simulink model "torqueBalancingSOT2017a"  (Simulink 8.9)
settings: Solver=FixedStepDiscrete  StartTime=0.0  StopTime=CONFIG.SIMULATION_TIME  FixedStep=CONFIG.Ts  RelTol=1e-3  EnableMultiTasking=on
InitFcn:
  | cd(fileparts(which(bdroot)));
  | initTorqueBalancingSOT;
undefined symbols (not defined in the file or in its folder): CONFIG, ConstraintsFeetMatrix, DiscIntNeverNeededParam, gain, reg, ROBOT_DOF, sat, sm, WBT_robotName
undefined symbols (not defined in the file): FRAMES
libraries: WBToolboxLibrary x76
(part 2 of 2)

== system torqueBalancingSOT2017a/Visualize and log/Visualize feet constraints ==
  wrench_leftFoot : Inport
  wrench_rightFoot : Inport  Port=2
  feetConstraints : Inport  Port=3
  state : Inport  Port=4
  Enable : EnablePort
  Feet Constraints : Scope  NumInputPorts=4
  wires:
  state/1 -> Feet Constraints/4  "state"
  feetConstraints/1 -> Feet Constraints/3  "feetConstraints"
  wrench_rightFoot/1 -> Feet Constraints/2  "wrench_rightFoot"
  wrench_leftFoot/1 -> Feet Constraints/1  "wrench_leftFoot"

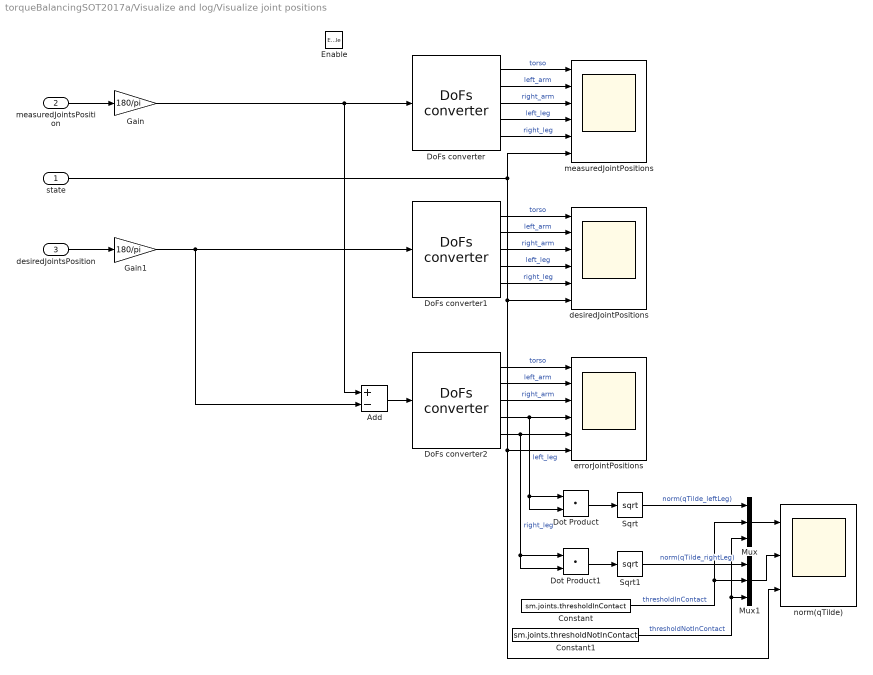
== system torqueBalancingSOT2017a/Visualize and log/Visualize joint positions ==
  state : Inport
  measuredJointsPosition : Inport  Port=2
  desiredJointsPosition : Inport  Port=3
  Enable : EnablePort
  Add : Sum  Inputs=+-
  Constant : Constant  Value=sm.joints.thresholdInContact
  Constant1 : Constant  Value=sm.joints.thresholdNotInContact
  DoFs converter : WBToolboxLibrary/Utilities/DoFs converter  yarp2WBIOption=From WBI to YARP  robotName=WBT_robotName  localName=WBT_modelName  wbiFile=WBT_wbiFilename  wbiList=WBT_wbiList
      settings: SourceProductName=Whole Body Toolbox
  DoFs converter1 : WBToolboxLibrary/Utilities/DoFs converter  yarp2WBIOption=From WBI to YARP  robotName=WBT_robotName  localName=WBT_modelName  wbiFile=WBT_wbiFilename  wbiList=WBT_wbiList
      settings: SourceProductName=Whole Body Toolbox
  DoFs converter2 : WBToolboxLibrary/Utilities/DoFs converter  yarp2WBIOption=From WBI to YARP  robotName=WBT_robotName  localName=WBT_modelName  wbiFile=WBT_wbiFilename  wbiList=WBT_wbiList
      settings: SourceProductName=Whole Body Toolbox
  Dot Product : DotProduct  InputSameDT=on  OutDataTypeStr=Inherit: Inherit via internal rule
  Dot Product1 : DotProduct  InputSameDT=on  OutDataTypeStr=Inherit: Inherit via internal rule
  Gain : Gain  Gain=180/pi
  Gain1 : Gain  Gain=180/pi
  Mux : Mux  Inputs=3
  Mux1 : Mux  Inputs=3
  Sqrt : Sqrt  SaturateOnIntegerOverflow=on
  Sqrt1 : Sqrt  SaturateOnIntegerOverflow=on
  desiredJointPositions : Scope  NumInputPorts=6
  errorJointPositions : Scope  NumInputPorts=6
  measuredJointPositions : Scope  NumInputPorts=6
  norm(qTilde) : Scope  NumInputPorts=3
  wires:
  DoFs converter/5 -> measuredJointPositions/5  "right_leg"
  DoFs converter/4 -> measuredJointPositions/4  "left_leg"
  DoFs converter/2 -> measuredJointPositions/2  "left_arm"
  DoFs converter/1 -> measuredJointPositions/1  "torso"
  DoFs converter2/2 -> errorJointPositions/2  "left_arm"
  DoFs converter2/1 -> errorJointPositions/1  "torso"
  desiredJointsPosition/1 -> Gain1/1
  measuredJointsPosition/1 -> Gain/1
  DoFs converter2/4 -> errorJointPositions/4, Dot Product/1, Dot Product/2  "left_leg"
  DoFs converter1/1 -> desiredJointPositions/1  "torso"
  DoFs converter1/3 -> desiredJointPositions/3  "right_arm"
  DoFs converter1/4 -> desiredJointPositions/4  "left_leg"
  Add/1 -> DoFs converter2/1
  Gain/1 -> Add/1, DoFs converter/1
  DoFs converter/3 -> measuredJointPositions/3  "right_arm"
  DoFs converter1/2 -> desiredJointPositions/2  "left_arm"
  DoFs converter2/3 -> errorJointPositions/3  "right_arm"
  DoFs converter2/5 -> errorJointPositions/5, Dot Product1/2, Dot Product1/1  "right_leg"
  DoFs converter1/5 -> desiredJointPositions/5  "right_leg"
  state/1 -> measuredJointPositions/6, norm(qTilde)/3, errorJointPositions/6, desiredJointPositions/6
  Dot Product/1 -> Sqrt/1
  Dot Product1/1 -> Sqrt1/1
  Sqrt/1 -> Mux/1  "norm(qTilde_leftLeg)"
  Sqrt1/1 -> Mux1/1  "norm(qTilde_rightLeg)"
  Constant/1 -> Mux/2, Mux1/2  "thresholdInContact"
  Constant1/1 -> Mux1/3, Mux/3  "thresholdNotInContact"
  Mux/1 -> norm(qTilde)/1
  Mux1/1 -> norm(qTilde)/2
  Gain1/1 -> Add/2, DoFs converter1/1

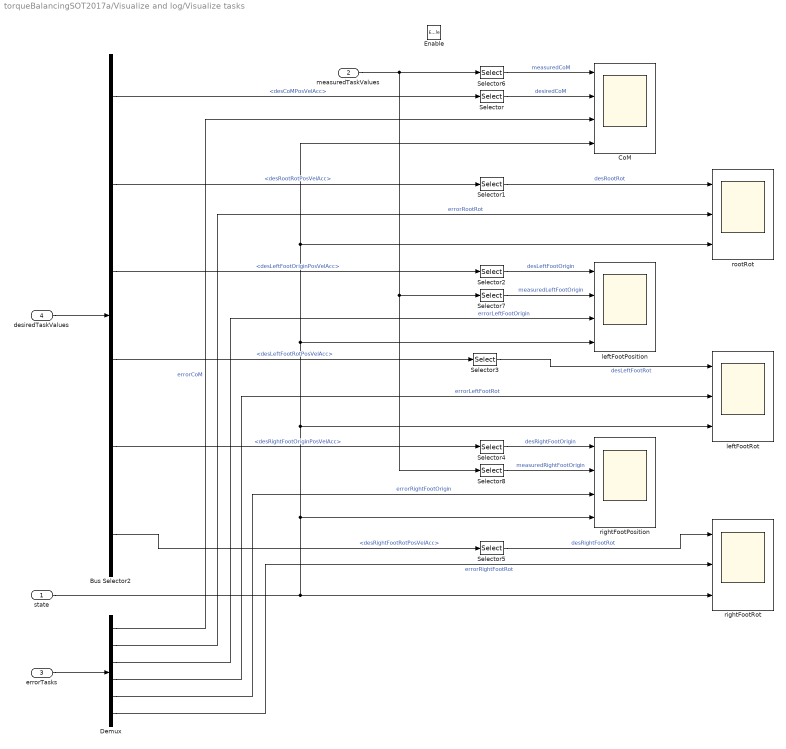
== system torqueBalancingSOT2017a/Visualize and log/Visualize tasks ==
  state : Inport
  measuredTaskValues : Inport  Port=2
  errorTasks : Inport  Port=3
  desiredTaskValues : Inport  Port=4
  Enable : EnablePort
  Bus Selector2 : BusSelector  OutputSignals=desCoMPosVelAcc,desRootRotPosVelAcc,desLeftFootOriginPosVelAcc,desLeftFootRotPosVelAcc,desRightFootOriginPosVelAcc,desRightFootRotPosVelAcc
  CoM : Scope  NumInputPorts=4
  Demux : Demux  Outputs=6
  Selector : Selector  NumberOfDimensions=2  InputPortWidth=9  IndexOptions=Index vector (dialog),Index vector (dialog)  Indices=[1:3],1  OutputSizes=1,1
  Selector1 : Selector  NumberOfDimensions=2  InputPortWidth=9  IndexOptions=Index vector (dialog),Index vector (dialog)  Indices=[1:3],[1:3]  OutputSizes=1,1
  Selector2 : Selector  NumberOfDimensions=2  InputPortWidth=9  IndexOptions=Index vector (dialog),Index vector (dialog)  Indices=[1:3],1  OutputSizes=1,1
  Selector3 : Selector  NumberOfDimensions=2  InputPortWidth=9  IndexOptions=Index vector (dialog),Index vector (dialog)  Indices=[1:3],[1:3]  OutputSizes=1,1
  Selector4 : Selector  NumberOfDimensions=2  InputPortWidth=9  IndexOptions=Index vector (dialog),Index vector (dialog)  Indices=[1:3],1  OutputSizes=1,1
  Selector5 : Selector  NumberOfDimensions=2  InputPortWidth=9  IndexOptions=Index vector (dialog),Index vector (dialog)  Indices=[1:3],[1:3]  OutputSizes=1,1
  Selector6 : Selector  NumberOfDimensions=2  InputPortWidth=9  IndexOptions=Index vector (dialog),Index vector (dialog)  Indices=[1:3],4  OutputSizes=1,1
  Selector7 : Selector  NumberOfDimensions=2  InputPortWidth=9  IndexOptions=Index vector (dialog),Index vector (dialog)  Indices=[5:8],4  OutputSizes=1,1
  Selector8 : Selector  NumberOfDimensions=2  InputPortWidth=9  IndexOptions=Index vector (dialog),Index vector (dialog)  Indices=[9:11],4  OutputSizes=1,1
  leftFootPosition : Scope  NumInputPorts=4
  leftFootRot : Scope  NumInputPorts=3
  rightFootPosition : Scope  NumInputPorts=4
  rightFootRot : Scope  NumInputPorts=3
  rootRot : Scope  NumInputPorts=3
  wires:
  Selector/1 -> CoM/2  "desiredCoM"
  Demux/1 -> CoM/3  "errorCoM"
  state/1 -> CoM/4, rootRot/3, leftFootPosition/4, leftFootRot/3, rightFootPosition/4, rightFootRot/3
  Selector6/1 -> CoM/1  "measuredCoM"
  Demux/3 -> leftFootPosition/3  "errorLeftFootOrigin"
  Demux/5 -> rightFootPosition/3  "errorRightFootOrigin"
  Selector2/1 -> leftFootPosition/1  "desLeftFootOrigin"
  Selector7/1 -> leftFootPosition/2  "measuredLeftFootOrigin"
  Selector4/1 -> rightFootPosition/1  "desRightFootOrigin"
  Selector8/1 -> rightFootPosition/2  "measuredRightFootOrigin"
  Selector1/1 -> rootRot/1  "desRootRot"
  Selector3/1 -> leftFootRot/1  "desLeftFootRot"
  Selector5/1 -> rightFootRot/1  "desRightFootRot"
  Demux/2 -> rootRot/2  "errorRootRot"
  Demux/4 -> leftFootRot/2  "errorLeftFootRot"
  Demux/6 -> rightFootRot/2  "errorRightFootRot"
  measuredTaskValues/1 -> Selector8/1, Selector7/1, Selector6/1
  errorTasks/1 -> Demux/1
  Bus Selector2/4 -> Selector3/1  "<desLeftFootRotPosVelAcc>"
  Bus Selector2/6 -> Selector5/1  "<desRightFootRotPosVelAcc>"
  Bus Selector2/2 -> Selector1/1  "<desRootRotPosVelAcc>"
  desiredTaskValues/1 -> Bus Selector2/1
  Bus Selector2/1 -> Selector/1  "<desCoMPosVelAcc>"
  Bus Selector2/3 -> Selector2/1  "<desLeftFootOriginPosVelAcc>"
  Bus Selector2/5 -> Selector4/1  "<desRightFootOriginPosVelAcc>"

== system torqueBalancingSOT2017a/Visualize and log/Visualize torques ==
  state : Inport
  measuredJointsTorque : Inport  Port=2
  desiredJointsTorque : Inport  Port=3
  Enable : EnablePort
  Add : Sum  Inputs=+-
  DoFs converter : WBToolboxLibrary/Utilities/DoFs converter  yarp2WBIOption=From WBI to YARP  robotName=WBT_robotName  localName=WBT_modelName  wbiFile=WBT_wbiFilename  wbiList=WBT_wbiList
      settings: SourceProductName=Whole Body Toolbox
  DoFs converter1 : WBToolboxLibrary/Utilities/DoFs converter  yarp2WBIOption=From WBI to YARP  robotName=WBT_robotName  localName=WBT_modelName  wbiFile=WBT_wbiFilename  wbiList=WBT_wbiList
      settings: SourceProductName=Whole Body Toolbox
  DoFs converter2 : WBToolboxLibrary/Utilities/DoFs converter  yarp2WBIOption=From WBI to YARP  robotName=WBT_robotName  localName=WBT_modelName  wbiFile=WBT_wbiFilename  wbiList=WBT_wbiList
      settings: SourceProductName=Whole Body Toolbox
  desiredJointTorques : Scope  NumInputPorts=6
  errorJointTorques : Scope  NumInputPorts=6
  measuredJointTorques : Scope  NumInputPorts=6
  wires:
  DoFs converter1/2 -> desiredJointTorques/2  "left_arm"
  DoFs converter2/3 -> errorJointTorques/3  "right_arm"
  DoFs converter2/5 -> errorJointTorques/5  "right_leg"
  DoFs converter2/1 -> errorJointTorques/1  "torso"
  DoFs converter/5 -> measuredJointTorques/5  "right_leg"
  DoFs converter/4 -> measuredJointTorques/4  "left_leg"
  DoFs converter/2 -> measuredJointTorques/2  "left_arm"
  DoFs converter/1 -> measuredJointTorques/1  "torso"
  desiredJointsTorque/1 -> DoFs converter1/1, Add/2
  measuredJointsTorque/1 -> Add/1, DoFs converter/1
  DoFs converter/3 -> measuredJointTorques/3  "right_arm"
  DoFs converter2/4 -> errorJointTorques/4  "left_leg"
  DoFs converter1/1 -> desiredJointTorques/1  "torso"
  DoFs converter1/3 -> desiredJointTorques/3  "right_arm"
  DoFs converter1/4 -> desiredJointTorques/4  "left_leg"
  DoFs converter2/2 -> errorJointTorques/2  "left_arm"
  Add/1 -> DoFs converter2/1
  DoFs converter1/5 -> desiredJointTorques/5  "right_leg"
  state/1 -> measuredJointTorques/6, errorJointTorques/6, desiredJointTorques/6

== system torqueBalancingSOT2017a/synchronizer/GAZEBO_SYNCHRONIZER ==
  Enable : EnablePort
  Simulator Synchronizer : WBToolboxLibrary/Utilities/Simulator Synchronizer  period=CONFIG.Ts  serverPortName='/clock/rpc'  clientPortName='/WBT_synchronizer/rpc:o'
      settings: SourceProductName=Whole Body Toolbox

== system torqueBalancingSOT2017a/synchronizer/REAL_TIME_SYNC ==
  Enable : EnablePort
  Real Time Synchronizer : WBToolboxLibrary/Utilities/Real Time Synchronizer  period=CONFIG.Ts
      settings: SourceProductName=Whole Body Toolbox

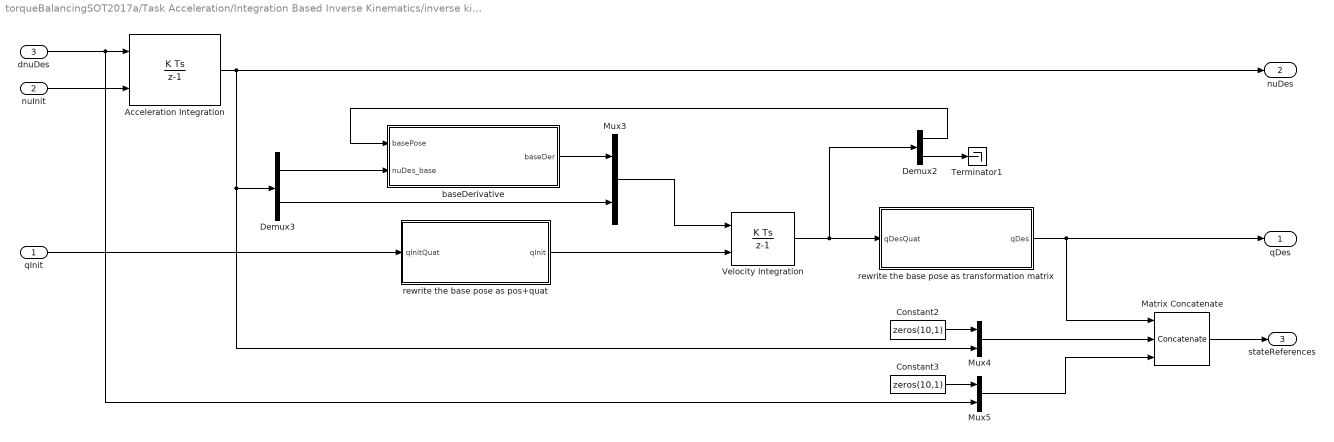
== system torqueBalancingSOT2017a/Task Acceleration/Integration Based Inverse Kinematics/inverse kinematics integration ==
  qInit : Inport
  nuInit : Inport  Port=2
  dnuDes : Inport  Port=3
  Acceleration Integration : DiscreteIntegrator  InitialConditionSource=external  SampleTime=CONFIG.Ts  ICPrevOutput=DiscIntNeverNeededParam  ICPrevScaledInput=DiscIntNeverNeededParam
  Constant2 : Constant  Value=zeros(10,1)
  Constant3 : Constant  Value=zeros(10,1)
  Demux2 : Demux  Outputs=[7;ROBOT_DOF]
  Demux3 : Demux  Outputs=[6;ROBOT_DOF]
  Matrix Concatenate : Concatenate  NumInputs=3  Mode=Multidimensional array  ConcatenateDimension=2
  Mux3 : Mux  Inputs=2
  Mux4 : Mux  Inputs=2
  Mux5 : Mux  Inputs=2
  Terminator1 : Terminator
  Velocity Integration : DiscreteIntegrator  InitialConditionSource=external  SampleTime=CONFIG.Ts  ICPrevOutput=DiscIntNeverNeededParam  ICPrevScaledInput=DiscIntNeverNeededParam
  baseDerivative : MATLAB Function  TreatAsAtomicUnit=on
  rewrite the base pose as pos+quat : MATLAB Function  TreatAsAtomicUnit=on
  rewrite the base pose as transformation matrix : MATLAB Function  TreatAsAtomicUnit=on
  qDes : Outport
  nuDes : Outport  Port=2
  stateReferences : Outport  Port=3
  wires:
  nuInit/1 -> Acceleration Integration/2
  qInit/1 -> rewrite the base pose as pos+quat/1(qInitQuat)
  dnuDes/1 -> Mux5/2, Acceleration Integration/1
  Demux2/2 -> Terminator1/1
  Demux2/1 -> baseDerivative/1(basePose)
  Velocity Integration/1 -> Demux2/1, rewrite the base pose as transformation matrix/1(qDesQuat)
  Acceleration Integration/1 -> Mux4/2, Demux3/1, nuDes/1
  Demux3/1 -> baseDerivative/2(nuDes_base)
  baseDerivative/1(baseDer) -> Mux3/1
  Demux3/2 -> Mux3/2
  Mux3/1 -> Velocity Integration/1
  Matrix Concatenate/1 -> stateReferences/1
  rewrite the base pose as transformation matrix/1(qDes) -> Matrix Concatenate/1, qDes/1
  rewrite the base pose as pos+quat/1(qInit) -> Velocity Integration/2
  Constant2/1 -> Mux4/1
  Mux4/1 -> Matrix Concatenate/2
  Constant3/1 -> Mux5/1
  Mux5/1 -> Matrix Concatenate/3

== system torqueBalancingSOT2017a/Task Acceleration/Integration Based Inverse Kinematics/referenceAccelerations ==
  qDes : Inport
  nuDes : Inport  Port=2
  desTaskValues : Inport  Port=3
  desJointAngles : Inport  Port=4
  impedances : Inport  Port=5
  dampings : Inport  Port=6
  PDgainsPos : Inport  Port=7
  PDgainsRot : Inport  Port=8
  Demux : Demux  Outputs=[16;ROBOT_DOF]
  Demux1 : Demux  Outputs=[6;ROBOT_DOF]
  Jacobians : Subsystem
  Kinematics : Subsystem
  Reshape : Reshape  OutputDimensionality=Customize  OutputDimensions=[4,4]
  Task and Joint Accelerations : Subsystem
  trajectoryGeneratorCoM2 : MATLAB Function  TreatAsAtomicUnit=on
  dnuDes : Outport
  wires:
  Demux/1 -> Reshape/1
  Demux1/2 -> Jacobians/4(jointVelocity), Task and Joint Accelerations/2(jointVelocities)
  qDes/1 -> Demux/1
  Reshape/1 -> Kinematics/1(w_H_b), Jacobians/1(w_H_b)
  Demux/2 -> Kinematics/2(JointAngles), Task and Joint Accelerations/4(jointAngles), Jacobians/2(JointAngles)
  trajectoryGeneratorCoM2/1(dnuDes) -> dnuDes/1
  nuDes/1 -> Demux1/1, Task and Joint Accelerations/3(nuDes)
  Jacobians/1(Jtask) -> Task and Joint Accelerations/1(Jtask), trajectoryGeneratorCoM2/1(Jtask)
  Jacobians/2(dJNu_task) -> trajectoryGeneratorCoM2/2(dJnuDes)
  Demux1/1 -> Jacobians/3(baseVelocity)
  desJointAngles/1 -> Task and Joint Accelerations/5(desJointAngles)
  desTaskValues/1 -> Task and Joint Accelerations/7(desTaskValues)
  Task and Joint Accelerations/2(jointsAccelerations) -> trajectoryGeneratorCoM2/4(jointDynamics)
  Task and Joint Accelerations/1(desTaskAcc) -> trajectoryGeneratorCoM2/3(taskAccelerations)
  impedances/1 -> Task and Joint Accelerations/8(impedances)
  dampings/1 -> Task and Joint Accelerations/9(dampings)
  PDgainsPos/1 -> Task and Joint Accelerations/10(PDgainsPos)
  PDgainsRot/1 -> Task and Joint Accelerations/11(PDgainsRot)
  Kinematics/1(taskPos) -> Task and Joint Accelerations/6(task_pos)

== system torqueBalancingSOT2017a/Task Acceleration/Integration Based Inverse Kinematics/referenceAccelerations/Jacobians ==
  w_H_b : Inport
  JointAngles : Inport  Port=2
  baseVelocity : Inport  Port=3
  jointVelocity : Inport  Port=4
  DotJ Nu : WBToolboxLibrary/wholeBodyModel/Jacobians/DotJ Nu  frameName='com'  robotName=WBT_robotName  localName=WBT_modelName  wbiFile=WBT_wbiFilename  wbiList=WBT_wbiList
      settings: SourceProductName=Whole Body Toolbox
  DotJ Nu1 : WBToolboxLibrary/wholeBodyModel/Jacobians/DotJ Nu  frameName='root_link'  robotName=WBT_robotName  localName=WBT_modelName  wbiFile=WBT_wbiFilename  wbiList=WBT_wbiList
      settings: SourceProductName=Whole Body Toolbox
  DotJ Nu2 : WBToolboxLibrary/wholeBodyModel/Jacobians/DotJ Nu  frameName='l_sole'  robotName=WBT_robotName  localName=WBT_modelName  wbiFile=WBT_wbiFilename  wbiList=WBT_wbiList
      settings: SourceProductName=Whole Body Toolbox
  DotJ Nu3 : WBToolboxLibrary/wholeBodyModel/Jacobians/DotJ Nu  frameName='r_sole'  robotName=WBT_robotName  localName=WBT_modelName  wbiFile=WBT_wbiFilename  wbiList=WBT_wbiList
      settings: SourceProductName=Whole Body Toolbox
  Jacobian1 : WBToolboxLibrary/wholeBodyModel/Jacobians/Jacobian  frameName='com'  robotName=WBT_robotName  localName=WBT_modelName  wbiFile=WBT_wbiFilename  wbiList=WBT_wbiList
      settings: SourceProductName=Whole Body Toolbox
  Jacobian2 : WBToolboxLibrary/wholeBodyModel/Jacobians/Jacobian  frameName='root_link'  robotName=WBT_robotName  localName=WBT_modelName  wbiFile=WBT_wbiFilename  wbiList=WBT_wbiList
      settings: SourceProductName=Whole Body Toolbox
  Jacobian3 : WBToolboxLibrary/wholeBodyModel/Jacobians/Jacobian  frameName='l_sole'  robotName=WBT_robotName  localName=WBT_modelName  wbiFile=WBT_wbiFilename  wbiList=WBT_wbiList
      settings: SourceProductName=Whole Body Toolbox
  Jacobian4 : WBToolboxLibrary/wholeBodyModel/Jacobians/Jacobian  frameName='r_sole'  robotName=WBT_robotName  localName=WBT_modelName  wbiFile=WBT_wbiFilename  wbiList=WBT_wbiList
      settings: SourceProductName=Whole Body Toolbox
  Matrix Concatenate1 : Concatenate  NumInputs=4  Mode=Multidimensional array
  Matrix Concatenate2 : Concatenate  NumInputs=4  Mode=Multidimensional array
  Selector2 : Selector  NumberOfDimensions=2  InputPortWidth=6+ROBOT_DOF  IndexOptions=Index vector (dialog),Index vector (dialog)  Indices=[4:6],[1:6+ROBOT_DOF]  OutputSizes=1,1
  Selector3 : Selector  NumberOfDimensions=2  InputPortWidth=6+ROBOT_DOF  IndexOptions=Index vector (dialog),Index vector (dialog)  Indices=[1:3],[1:6+ROBOT_DOF]  OutputSizes=1,1
  Selector4 : Selector  InputPortWidth=6  IndexOptions=Index vector (dialog)  Indices=[1:3]  OutputSizes=1
  Selector5 : Selector  InputPortWidth=6  IndexOptions=Index vector (dialog)  Indices=[4:6]  OutputSizes=1
  Jtask : Outport
  dJNu_task : Outport  Port=2
  wires:
  Jacobian1/1 -> Selector3/1
  jointVelocity/1 -> DotJ Nu1/4, DotJ Nu2/4, DotJ Nu3/4, DotJ Nu/4
  Jacobian2/1 -> Selector2/1
  Selector5/1 -> Matrix Concatenate2/2
  DotJ Nu2/1 -> Matrix Concatenate2/3
  Matrix Concatenate2/1 -> dJNu_task/1
  DotJ Nu3/1 -> Matrix Concatenate2/4
  Jacobian4/1 -> Matrix Concatenate1/4
  DotJ Nu/1 -> Selector4/1
  Selector4/1 -> Matrix Concatenate2/1
  Jacobian3/1 -> Matrix Concatenate1/3
  w_H_b/1 -> Jacobian1/1, Jacobian2/1, Jacobian3/1, Jacobian4/1, DotJ Nu/1, DotJ Nu1/1, DotJ Nu2/1, DotJ Nu3/1
  JointAngles/1 -> Jacobian2/2, Jacobian3/2, Jacobian4/2, DotJ Nu/2, DotJ Nu1/2, DotJ Nu2/2, DotJ Nu3/2, Jacobian1/2
  DotJ Nu1/1 -> Selector5/1
  baseVelocity/1 -> DotJ Nu/3, DotJ Nu1/3, DotJ Nu2/3, DotJ Nu3/3
  Selector3/1 -> Matrix Concatenate1/1
  Matrix Concatenate1/1 -> Jtask/1
  Selector2/1 -> Matrix Concatenate1/2

== system torqueBalancingSOT2017a/Task Acceleration/Integration Based Inverse Kinematics/referenceAccelerations/Kinematics ==
  w_H_b : Inport
  JointAngles : Inport  Port=2
  Forward KinematicsCoM : WBToolboxLibrary/wholeBodyModel/Kinematics/Forward Kinematics  frameName='com'  robotName=WBT_robotName  localName=WBT_modelName  wbiFile=WBT_wbiFilename  wbiList=WBT_wbiList
      settings: SourceProductName=Whole Body Toolbox
  Forward KinematicsCoM1 : WBToolboxLibrary/wholeBodyModel/Kinematics/Forward Kinematics  frameName='root_link'  robotName=WBT_robotName  localName=WBT_modelName  wbiFile=WBT_wbiFilename  wbiList=WBT_wbiList
      settings: SourceProductName=Whole Body Toolbox
  Forward Kinematics_lFoot : WBToolboxLibrary/wholeBodyModel/Kinematics/Forward Kinematics  frameName='l_sole'  robotName=WBT_robotName  localName=WBT_modelName  wbiFile=WBT_wbiFilename  wbiList=WBT_wbiList
      settings: SourceProductName=Whole Body Toolbox
  Forward Kinematics_rFoot : WBToolboxLibrary/wholeBodyModel/Kinematics/Forward Kinematics  frameName='r_sole'  robotName=WBT_robotName  localName=WBT_modelName  wbiFile=WBT_wbiFilename  wbiList=WBT_wbiList
      settings: SourceProductName=Whole Body Toolbox
  Matrix Concatenate : Concatenate  NumInputs=3  Mode=Multidimensional array
  Matrix Concatenate1 : Concatenate  Mode=Multidimensional array  ConcatenateDimension=2
  Selector : Selector  NumberOfDimensions=2  InputPortWidth=6+ROBOT_DOF  IndexOptions=Index vector (dialog),Index vector (dialog)  Indices=[1:4],[4]  OutputSizes=1,1
  Selector1 : Selector  NumberOfDimensions=2  InputPortWidth=6+ROBOT_DOF  IndexOptions=Index vector (dialog),Index vector (dialog)  Indices=[1:4],[1:3]  OutputSizes=1,1
  taskPos : Outport
  wires:
  JointAngles/1 -> Forward Kinematics_rFoot/2, Forward Kinematics_lFoot/2, Forward KinematicsCoM/2, Forward KinematicsCoM1/2
  w_H_b/1 -> Forward Kinematics_rFoot/1, Forward Kinematics_lFoot/1, Forward KinematicsCoM/1, Forward KinematicsCoM1/1
  Selector/1 -> Matrix Concatenate1/2
  Forward KinematicsCoM1/1 -> Selector1/1
  Selector1/1 -> Matrix Concatenate1/1
  Forward Kinematics_rFoot/1 -> Matrix Concatenate/3
  Forward KinematicsCoM/1 -> Selector/1
  Forward Kinematics_lFoot/1 -> Matrix Concatenate/2
  Matrix Concatenate/1 -> taskPos/1
  Matrix Concatenate1/1 -> Matrix Concatenate/1

== system torqueBalancingSOT2017a/Task Acceleration/Integration Based Inverse Kinematics/referenceAccelerations/Task and Joint Accelerations ==
  Jtask : Inport
  jointVelocities : Inport  Port=2
  nuDes : Inport  Port=3
  jointAngles : Inport  Port=4
  desJointAngles : Inport  Port=5
  task_pos : Inport  Port=6
  desTaskValues : Inport  Port=7
  impedances : Inport  Port=8
  dampings : Inport  Port=9
  PDgainsPos : Inport  Port=10
  PDgainsRot : Inport  Port=11
  Bus Selector : BusSelector  OutputSignals=desCoMPosVelAcc,desRootRotPosVelAcc,desLeftFootOriginPosVelAcc,desLeftFootRotPosVelAcc,desRightFootOriginPosVelAcc,desRightFootRotPosVelAcc
  Product : Product  Multiplication=Matrix(*)
  TaskAccelerations : MATLAB Function  TreatAsAtomicUnit=on
  jointAccelerations : MATLAB Function  TreatAsAtomicUnit=on
  desTaskAcc : Outport
  jointsAccelerations : Outport  Port=2
  wires:
  nuDes/1 -> Product/2
  Bus Selector/6 -> TaskAccelerations/8(desRFootRotPosVelAcc)  "<desRightFootRotPosVelAcc>"
  desTaskValues/1 -> Bus Selector/1
  Bus Selector/4 -> TaskAccelerations/6(desLFootRotPosVelAcc)  "<desLeftFootRotPosVelAcc>"
  jointAngles/1 -> jointAccelerations/1(jointAngles)
  Bus Selector/3 -> TaskAccelerations/5(desLFootOriginPosVelAcc)  "<desLeftFootOriginPosVelAcc>"
  Bus Selector/2 -> TaskAccelerations/4(desRootRotPosVelAcc)  "<desRootRotPosVelAcc>"
  TaskAccelerations/1(desiredTaskAcc) -> desTaskAcc/1
  Jtask/1 -> Product/1
  jointVelocities/1 -> jointAccelerations/3(jointVelocities)
  jointAccelerations/1(jointAccelerations) -> jointsAccelerations/1
  Bus Selector/5 -> TaskAccelerations/7(desRFootOriginPosVelAcc)  "<desRightFootOriginPosVelAcc>"
  desJointAngles/1 -> jointAccelerations/2(desJointAngles)
  Product/1 -> TaskAccelerations/2(taskVelocities)
  impedances/1 -> jointAccelerations/4(dampings)
  dampings/1 -> jointAccelerations/5(impedances)
  PDgainsPos/1 -> TaskAccelerations/9(PDgainsPos)
  PDgainsRot/1 -> TaskAccelerations/10(PDgainsRot)
  Bus Selector/1 -> TaskAccelerations/3(desComPosVelAcc)  "<desCoMPosVelAcc>"
  task_pos/1 -> TaskAccelerations/1(taskPositions)

== matlab function Task Acceleration/Integration Based Inverse Kinematics/referenceAccelerations/Task and Joint Accelerations/jointAccelerations ==
  data: jointAngles input double; desJointAngles input double; jointVelocities input double; jointAccelerations output double; dampings input double; impedances input double
function jointAccelerations = jointDynamicsFCN(jointAngles, desJointAngles, jointVelocities, dampings, impedances)
                            
jointAccelerations = jointDynamics(jointAngles, desJointAngles, jointVelocities, impedances, dampings);

== matlab function Desired values/stateMachineWalkingFCN ==
  data: qDes output double; qj input double; qj0 input double; CoM_0 input double; l_sole_CoM input double; r_sole_CoM input double; l_sole_H_b input double; r_sole_H_b input double; rotFrame_H_b0 input double; wrench_leftFoot input double; wrench_rightFoot input double; CoMDes output double; desRootRotPosVelAcc output double; desLeftFootOriginPos output double; desLeftFootRotPosVelAcc output double; desRightFootOriginPos output double; desRightFootRotPosVelAcc output double; impedances output double; dampings output double; PDgainsPos output double; PDgainsRot output double; jointsSmoothingTime output double; w_H_b output double; feetActivation output double; currentState output double; sm parameter double; gain parameter double; CONFIG parameter double
function [qDes, CoMDes, desRootRotPosVelAcc, ...
          desLeftFootOriginPos, desLeftFootRotPosVelAcc, desRightFootOriginPos, desRightFootRotPosVelAcc,  ...
          impedances, dampings, PDgainsPos, PDgainsRot, jointsSmoothingTime, w_H_b, feetActivation, currentState] ...
          = stateMachineWalkingFCN(qj, qj0, CoM_0, ...
                                   l_sole_CoM, r_sole_CoM, l_sole_H_b, r_sole_H_b, rotFrame_H_b0, ...
                                   wrench_leftFoot, wrench_rightFoot, sm, gain, CONFIG)

[w_H_b, CoMDes, qDes, feetActivation, impedances, dampings, PDgainsPos, PDgainsRot, currentState, jointsSmoothingTime,...
 desRootRotPosVelAcc, desLeftFootRotPosVelAcc, desLeftFootOriginPos, desRightFootRotPosVelAcc, desRightFootOriginPos] ...
= stateMachineWalking(qj, qj0, CoM_0, ...
                      l_sole_CoM, r_sole_CoM, l_sole_H_b, r_sole_H_b, rotFrame_H_b0, ...
                      wrench_leftFoot, wrench_rightFoot, sm, gain, CONFIG);

== matlab function Dynamics, Kinematics, Jacobians/Jacobians/baseVelocityFCN ==
  data: JcLeftFoot input double; vb output double; JcRightFoot input double; feetConstraints input double; dqj input double; reg parameter double
function vb = baseVelocityFCN(JcLeftFoot, JcRightFoot, feetConstraints, dqj, reg)

vb = baseVelocity(JcLeftFoot, JcRightFoot, feetConstraints, dqj, reg);

== matlab function Desired values/w_H_root_link2/fromImuToHomogeousTransformFCN ==
  data: imu_H_link input double; imu_H_link_0 input double; link_H_root input double; inertial_0 input double; inertial input double; neck input double; w_H_root output double; CONFIG parameter double
function w_H_root = fromBaseToWorldWithImuFCN(imu_H_link,imu_H_link_0,link_H_root,inertial_0,inertial,neck,CONFIG)
%#codegen
w_H_root = fromBaseToWorldWithImu(imu_H_link,imu_H_link_0,link_H_root,inertial_0,inertial,neck,CONFIG);

== matlab function Task Acceleration/Integration Based Inverse Kinematics/referenceAccelerations/Task and Joint Accelerations/TaskAccelerations ==
  data: taskPositions input double; taskVelocities input double; desComPosVelAcc input double; desiredTaskAcc output double; desRootRotPosVelAcc input double; desLFootOriginPosVelAcc input double; desLFootRotPosVelAcc input double; desRFootOriginPosVelAcc input double; desRFootRotPosVelAcc input double; PDgainsPos input double; PDgainsRot input double
function desiredTaskAcc   = desiredTaskAccelerationFCN...
         (taskPositions, taskVelocities, ...
                                      desComPosVelAcc, desRootRotPosVelAcc, ...
                                      desLFootOriginPosVelAcc, desLFootRotPosVelAcc, ...
                                      desRFootOriginPosVelAcc, desRFootRotPosVelAcc, ...
                                      PDgainsPos, PDgainsRot)     
     
     [desiredTaskAcc,~,~,~,~,~,~,~] = desiredTaskAcceleration(taskPositions, taskVelocities, ...
                                      desComPosVelAcc, desRootRotPosVelAcc, ...
                                      desLFootOriginPosVelAcc, desLFootRotPosVelAcc, ...
                                      desRFootOriginPosVelAcc, desRFootRotPosVelAcc, ...
                                      PDgainsPos, PDgainsRot);
                                            
end

== matlab function Task Acceleration/Desired task accelerations/desiredTaskAcceleration ==
  data: taskPositions input double; taskVelocities input double; desComPosVelAcc input double; desRootRotPosVelAcc input double; desLFootOriginPosVelAcc input double; desLFootRotPosVelAcc input double; desRFootOriginPosVelAcc input double; desRFootRotPosVelAcc input double; PDgainsPos input double; PDgainsRot input double; desiredTaskAcc output double; taskError output double
function [desiredTaskAcc, taskError] = ...
    desiredTaskAccelerationFCN(taskPositions, taskVelocities, ...
                                      desComPosVelAcc, desRootRotPosVelAcc, ...
                                      desLFootOriginPosVelAcc, desLFootRotPosVelAcc, ...
                                      desRFootOriginPosVelAcc, desRFootRotPosVelAcc, ...
                                      PDgainsPos, PDgainsRot)
    %[desiredTaskAcc, rootRotError, leftFootOriginError, leftFootRotError, rightFootOriginError, rightFootRotError]                                                 
                           
 [desiredTaskAcc, ~, ~, ~, ~, ~, ~, taskError] = ...
              desiredTaskAcceleration(taskPositions, taskVelocities, ...
                                      desComPosVelAcc, desRootRotPosVelAcc, ...
                                      desLFootOriginPosVelAcc, desLFootRotPosVelAcc, ...
                                      desRFootOriginPosVelAcc, desRFootRotPosVelAcc, ...
                                      PDgainsPos, PDgainsRot);

== matlab function Controller and QP/balancingController ==
  data: feetActivation input double; massMatrix input double; biasTorques input double; jacobiansDotNu input double; poseLeftFoot input double; poseRightFoot input double; jacobians input double; desJointAcc input double; hessianMatrix output double; desiredTaskAcc input double; ROBOT_DOF parameter double; ConstraintsMatrix input double; gain parameter double; CONFIG parameter double; biasVector output double; constraintMatrixLeftFoot output double; constraintMatrixRightFoot output double; constraintMatrixEq output double; upperBoundEqConstraints output double
function [hessianMatrix,biasVector,constraintMatrixLeftFoot,constraintMatrixRightFoot,constraintMatrixEq, upperBoundEqConstraints] = ...
                                        balancingControllerSOTFCN(feetActivation, ...
                                                               massMatrix, biasTorques, jacobiansDotNu, poseLeftFoot, poseRightFoot, jacobians, ...
                                                               desJointAcc, desiredTaskAcc, ...
                                                               ROBOT_DOF, ConstraintsMatrix, ...
                                                               gain, CONFIG)

[hessianMatrix,biasVector,constraintMatrixLeftFoot,constraintMatrixRightFoot,constraintMatrixEq, upperBoundEqConstraints] = ...
                                        balancingControllerSOT(feetActivation, ...
                                                               massMatrix, biasTorques, jacobiansDotNu, poseLeftFoot, poseRightFoot, jacobians, ...
                                                               desJointAcc, desiredTaskAcc, ...
                                                               ROBOT_DOF, ConstraintsMatrix, ...
                                                               gain, CONFIG);

== matlab function Task Acceleration/Integration Based Inverse Kinematics/referenceAccelerations/trajectoryGeneratorCoM2 ==
  data: Jtask input double; dJnuDes input double; taskAccelerations input double; jointDynamics input double; dnuDes output double; ROBOT_DOF parameter double; reg parameter double
function dnuDes   = referenceAccelerationFCN(Jtask, dJnuDes, taskAccelerations, jointDynamics, ... 
                                                      ROBOT_DOF, reg)
                                          
dnuDes   = referenceAcceleration(Jtask, dJnuDes, taskAccelerations, jointDynamics, ... 
                                 ROBOT_DOF, reg);

== matlab function Task Acceleration/jointAccelerations ==
  data: desJointAngles input double; jointAngles input double; robotVelocity input double; impedances input double; desJointAcc output double; dampings input double; ROBOT_DOF parameter double
function desJointAcc = fcn(desJointAngles, jointAngles, robotVelocity, impedances, dampings, ROBOT_DOF)

%     desJointAcc               = - diag(impedances)*(jointAngles-desJointAngles)...
%                                 - diag(dampings)  *robotVelocity(7:end);
desJointAcc = linearPID(jointAngles, robotVelocity(7:end), [desJointAngles zeros(ROBOT_DOF, 2)], [impedances dampings]);

== matlab function Task Acceleration/Integration Based Inverse Kinematics/inverse kinematics integration/baseDerivative ==
  data: basePose input double; nuDes_base input double; baseDer output double
function baseDer   = baseDerivative(basePose, nuDes_base)

% Time derivative of the floating base pose. The base orientation is in quaternions
baseDer            = baseDerivative(nuDes_base,basePose);

end

== matlab function Task Acceleration/Integration Based Inverse Kinematics/inverse kinematics integration/rewrite the base pose as pos+quat ==
  data: qInitQuat input double; qInit output double
function qInit = transfMatrixToQuaternions(qInitQuat)

% Converts the floating base in the initial state vector [16+ndof;1] to 
% position + quaternion representation 
qInit = transfMatrixToQuaternions(qInitQuat);

end

== matlab function Task Acceleration/Integration Based Inverse Kinematics/inverse kinematics integration/rewrite the base pose as transformation matrix ==
  data: qDesQuat input double; qDes output double
function qDes = fromQuaternionsToTransfMatr(qDesQuat)

% Converts the floating base pose from a quaternion representation to a 
% tranformation matrix
qDes = fromQuaternionsToTransfMatr(qDesQuat);

end

== matlab function Desired values/w_H_root_link1/fromImuToHomogeousTransformFCN ==
  data: imu_H_link input double; imu_H_link_0 input double; link_H_root input double; inertial_0 input double; inertial input double; neck input double; w_H_root output double; CONFIG parameter double
function w_H_root = fromBaseToWorldWithImuFCN(imu_H_link,imu_H_link_0,link_H_root,inertial_0,inertial,neck,CONFIG)
%#codegen
w_H_root = fromBaseToWorldWithImu(imu_H_link,imu_H_link_0,link_H_root,inertial_0,inertial,neck,CONFIG);

== matlab function Desired values/w_H_root_link4/fromImuToHomogeousTransformFCN ==
  data: imu_H_link input double; imu_H_link_0 input double; link_H_root input double; inertial_0 input double; inertial input double; neck input double; w_H_root output double; CONFIG parameter double
function w_H_root = fromBaseToWorldWithImuFCN(imu_H_link,imu_H_link_0,link_H_root,inertial_0,inertial,neck,CONFIG)
%#codegen
w_H_root = fromBaseToWorldWithImu(imu_H_link,imu_H_link_0,link_H_root,inertial_0,inertial,neck,CONFIG);
